simulink model "SalientPolePMSM"  (R2020b)
settings: Solver=VariableStepAuto  StartTime=0  StopTime=1  MaxStep=1e-4  RelTol=1e-4
values from neighbouring files (symbols this model uses):
  Bgain = 1    [DataSalientPolePMSM-DESKTOP-IINSHMA.m]    (also in DataSalientPolePMSM.m)
  Gcc_1ord = 1/(s/bandwidth(Gcc) + 1)    [DataSalientPolePMSM-DESKTOP-IINSHMA.m]    (also in DataSalientPolePMSM.m)
  lamdVec = mot.Ld*idVec+mot.lammg    [DataSalientPolePMSM-DESKTOP-IINSHMA.m]    (also in DataSalientPolePMSM.m)
  lamqVec = mot.Lq*iqVec    [DataSalientPolePMSM-DESKTOP-IINSHMA.m]    (also in DataSalientPolePMSM.m)
  TAB0_abc = Tabc_AB0^-1    [DataSalientPolePMSM-DESKTOP-IINSHMA.m]    (also in DataSalientPolePMSM.m)
  Tabc_AB0 = 2/3.*[     1       -1/2       -1/2 ... (first row only)    [DataSalientPolePMSM-DESKTOP-IINSHMA.m]    (also in DataSalientPolePMSM.m)
  Talphabeta_abc = Tabc_alphabeta^(-1)    [DataSalientPolePMSM-DESKTOP-IINSHMA.m]    (also in DataSalientPolePMSM.m)
undefined symbols (not defined in the file or in its folder): DiscIntNeverNeededParam, dqpll, inv, kid, kpd, magnitude, meas, mot, Obs, PI, stconv
libraries: simulink x53, pid_lib x3, powerlib x2, eeBldcCommutationLogic x1, electricdrivelib x1
(part 4 of 7)

== system SalientPolePMSM/DT SENSORLESS ALGORITHM AB/PII ==
  e : Inport
  Add : Sum  Inputs=+++
  Delay : Delay  DelayLength=1
  Delay1 : Delay  DelayLength=1
  Delay2 : Delay  DelayLength=1
  Discrete Filter1 : DiscreteFilter  Numerator=[Obs.lpf.alpha]  Denominator=[1 ((Obs.lpf.alpha)-1)]  SampleTime=Obs.Ts
  Discrete-Time Integrator : DiscreteIntegrator  SampleTime=Obs.Ts  ICPrevOutput=DiscIntNeverNeededParam  ICPrevScaledInput=DiscIntNeverNeededParam
  Gain1 : Gain  Gain=0.00001*0
  Gain6 : Gain  Gain=Obs.PI.ki*Obs.Ts*0.01
  Gain7 : Gain  Gain=Obs.PI.kp
  MATLAB Function1 : MATLAB Function  TreatAsAtomicUnit=on
  MATLAB Function2 : MATLAB Function  TreatAsAtomicUnit=on
  Sum1 : Sum  Inputs=++|
  Sum2 : Sum  Inputs=++|
  Sum3 : Sum  Inputs=++|
  w_est : Outport
  th_est : Outport  Port=2
  wires:
  Sum1/1 -> Delay/1
  Gain6/1 -> Add/1
  Delay/1 -> Gain6/1, Sum1/1
  Gain7/1 -> Add/2
  Delay1/1 -> Sum3/2, Sum2/1
  Sum2/1 -> Delay1/1
  Sum3/1 -> Delay2/1
  Delay2/1 -> Gain1/1, Sum3/1
  Gain1/1 -> Add/3
  Add/1 -> Discrete Filter1/1  "w_est"
  e/1 -> Sum2/2, Sum1/2, Gain7/1
  Discrete Filter1/1 -> Discrete-Time Integrator/1, MATLAB Function1/1(u)
  Discrete-Time Integrator/1 -> MATLAB Function2/1(u)
  MATLAB Function2/1(y) -> th_est/1
  MATLAB Function1/1(y) -> w_est/1

== system SalientPolePMSM/DT SENSORLESS ALGORITHM AB/Rev_Park + Rev_Clarke1 ==
  note: INPUTS
  Iabc : Inport
  Demux1 : Demux  Outputs=3
  Gain : Gain  Gain=sqrt(3)
  Gain1 : Gain  Gain=1/2
  Mux : Mux  Inputs=2
  Sum2 : Sum  Inputs=--|
  Terminator : Terminator
  AB : Outport
  wires:
  Demux1/3 -> Terminator/1
  Iabc/1 -> Demux1/1
  Demux1/2 -> Gain/1
  Gain/1 -> Sum2/2
  Sum2/1 -> Gain1/1
  Demux1/1 -> Mux/1, Sum2/1
  Mux/1 -> AB/1
  Gain1/1 -> Mux/2

== system SalientPolePMSM/DT SENSORLESS ALGORITHM AB/alpha axis observer ==
  u_alpha : Inport
  i_alpha_ref : Inport  Port=2
  wel_est : Inport  Port=3
  Gain : Gain  Gain=Obs.Ts/mot.Lq
  Gain1 : Gain  Gain=-mot.R*Obs.Ts/mot.Lq
  Gain2 : Gain  Gain=Obs.Lab(1)
  Gain3 : Gain  Gain=-Obs.Ts/mot.Lq
  Gain4 : Gain  Gain=Obs.Lab(2)
  Product : Product
  Sum{,1,3,5..6} (5 alike) : Sum  Inputs=|++
  Sum2 : Sum  Inputs=++|
  Sum4 : Sum  Inputs=-+|
  e_alpha(k+1) : Outport
  i_alpha(k + 1) : Outport  Port=2
  wires:
  Sum/1 -> Sum4/2, Sum/2, Gain1/1, i_alpha(k + 1)/1
  Gain/1 -> Sum3/1
  Gain1/1 -> Sum1/2
  Sum1/1 -> Sum/1
  i_alpha_ref/1 -> Sum4/1
  Sum4/1 -> Gain4/1, Gain2/1
  Gain2/1 -> Sum3/2
  Sum2/1 -> Sum1/1
  Sum3/1 -> Sum2/2
  Sum6/1 -> Gain3/1, Sum6/2, e_alpha(k+1)/1
  Gain3/1 -> Sum2/1
  Gain4/1 -> Sum5/2
  u_alpha/1 -> Product/2, Gain/1
  wel_est/1 -> Product/1
  Sum5/1 -> Sum6/1
  Product/1 -> Sum5/1

== system SalientPolePMSM/DT SENSORLESS ALGORITHM AB/alpha axis observer2 ==
  u_beta : Inport
  i_beta_ref : Inport  Port=2
  wel_est : Inport  Port=3
  Gain : Gain  Gain=Obs.Ts/mot.Lq
  Gain1 : Gain  Gain=-mot.R*Obs.Ts/mot.Lq
  Gain2 : Gain  Gain=Obs.Lab(1)
  Gain3 : Gain  Gain=-Obs.Ts/mot.Lq
  Gain4 : Gain  Gain=Obs.Lab(2)
  Product : Product
  Sum{,1,3,5..6} (5 alike) : Sum  Inputs=|++
  Sum2 : Sum  Inputs=++|
  Sum4 : Sum  Inputs=-+|
  e_beta(k+1) : Outport
  i_beta(k + 1) : Outport  Port=2
  wires:
  Sum/1 -> i_beta(k + 1)/1, Sum4/2, Sum/2, Gain1/1
  Gain/1 -> Sum3/1
  Gain1/1 -> Sum1/2
  Sum1/1 -> Sum/1
  i_beta_ref/1 -> Sum4/1
  Sum4/1 -> Gain4/1, Gain2/1
  Gain2/1 -> Sum3/2
  Sum2/1 -> Sum1/1
  Sum3/1 -> Sum2/2
  Sum5/1 -> Gain3/1, Sum5/2, e_beta(k+1)/1
  Gain3/1 -> Sum2/1
  Sum6/1 -> Sum5/1
  u_beta/1 -> Product/2, Gain/1
  Product/1 -> Sum6/1
  wel_est/1 -> Product/1
  Gain4/1 -> Sum6/2

== system SalientPolePMSM/DT SENSORLESS ALGORITHM DQ/Clarke + Park 5 ==
  note: INPUTS
  note: OUTPUT
  note: INPUTS
  abc : Inport
  thme : Inport  Port=2
  Add1 : Sum  Inputs=+-
  Add2 : Sum
  Add3 : Sum  Inputs=-+
  Add4 : Sum
  Cos1 : Trigonometry  Operator=cos
  Cos2 : Trigonometry  Operator=cos
  Demux1 : Demux  Outputs=3
  Demux2 : Demux  Outputs=3
  Demux3 : Demux  Outputs=3
  Gain : Gain  Gain=sqrt(3)
  Gain1 : Gain  Gain=Tabc_AB0  Multiplication=Matrix(K*u) (u vector)
  Gain10 : Gain  Gain=-1/sqrt(3)
  Gain2 : Gain  Gain=1/2
  Gain9 : Gain  Gain=2
  Mux : Mux  Inputs=2
  Mux1 : Mux  Inputs=2
  Mux2 : Mux  Inputs=3
  Product{,1..7} (8 alike) : Product
  Scope : Scope  NumInputPorts=2
  Sin1 : Trigonometry
  Sin2 : Trigonometry
  Sum2 : Sum  Inputs=--|
  Sum5 : Sum  Inputs=++|
  Terminator : Terminator
  Terminator1 : Terminator
  dq : Outport
  wires:
  Demux2/3 -> Terminator/1
  Product/1 -> Add2/1
  Product1/1 -> Add2/2
  Cos2/1 -> Product/2, Product3/1
  Demux2/1 -> Product3/2, Product1/1
  Product3/1 -> Add3/2
  Product2/1 -> Add3/1
  Demux2/2 -> Product2/1, Product/1
  Sin2/1 -> Product2/2, Product1/2
  Add3/1 -> Mux1/2
  Add2/1 -> Mux1/1
  Sum5/1 -> Gain10/1
  Gain9/1 -> Sum5/2
  Demux1/2 -> Gain9/1
  Demux1/3 -> Mux2/3
  Demux1/1 -> Mux2/1, Sum5/1
  Gain10/1 -> Mux2/2
  Gain1/1 -> Demux2/1, Scope/1
  Add1/1 -> Mux/1
  Sin1/1 -> Product5/2, Product4/2
  Gain/1 -> Sum2/2
  Product5/1 -> Add1/2
  Cos1/1 -> Product6/2, Product7/1
  Sum2/1 -> Gain2/1
  Demux3/1 -> Product5/1, Product6/1, Sum2/1
  Demux3/2 -> Gain/1
  Product4/1 -> Add4/2
  Product7/1 -> Add1/1
  Product6/1 -> Add4/1
  Demux3/3 -> Terminator1/1
  Add4/1 -> Mux/2
  Gain2/1 -> Product7/2, Product4/1
  thme/1 -> Sin2/1, Cos2/1
  Mux1/1 -> dq/1
  abc/1 -> Gain1/1

== system SalientPolePMSM/DT SENSORLESS ALGORITHM DQ/Classic PLL1 ==
  e_d : Inport
  e_q : Inport  Port=2
  Cos : Trigonometry  Operator=cos
  Delay{1..4} (4 alike) : Delay  DelayLength=1  SampleTime=Obs.Ts
  Discrete Filter1 : DiscreteFilter  Commented=on  Numerator=[dqpll.lpf.alpha]  Denominator=[1 (dqpll.lpf.alpha-1)]
  Discrete PID Controller : pid_lib/PID Controller  Controller=PID  Form=Parallel  TimeDomain=Discrete-time  UseExternalTs=off  SampleTime=Obs.Ts  IntegratorMethod=Forward Euler  FilterMethod=Forward Euler  ControllerParametersSource=internal  P=Obs.PI.kp*0.01  I=Obs.PI.ki*0.1  D=0  UseFilter=off  N=100  TunerSelectOption=Transfer Function Based (PID Tuner App)  ZeroCross=off  InitialConditionSource=internal  InitialConditionForIntegrator=0  InitialConditionForFilter=0  DifferentiatorICPrevScaledInput=0  ExternalReset=none  TrackingMode=off  Kt=1  LimitOutput=off  SatLimitsSource=internal  UpperSaturationLimit=inf  LowerSaturationLimit=-inf  LinearizeAsGain=off  AntiWindupMode=none  Kb=1  POutMin=[]  POutMax=[]  IOutMin=[]  IOutMax=[]  DOutMin=[]  DOutMax=[]  NOutMin=[]  NOutMax=[]  SumOutMin=[]  SumOutMax=[]  SaturationOutMin=[]  SaturationOutMax=[]  PParamMin=[]  PParamMax=[]  IParamMin=[]  IParamMax=[]  DParamMin=[]  DParamMax=[]  NParamMin=[]  NParamMax=[]  KbParamMin=[]  KbParamMax=[]  KtParamMin=[]  KtParamMax=[]  KbOutMin=[]  KbOutMax=[]  KtOutMin=[]  KtOutMax=[]  IntegratorOutMin=[]  IntegratorOutMax=[]  FilterOutMin=[]  FilterOutMax=[]  SumI1OutMin=[]  SumI1OutMax=[]  SumI2OutMin=[]  SumI2OutMax=[]  SumI3OutMin=[]  SumI3OutMax=[]  SumI4OutMin=[]  SumI4OutMax=[]  SumDOutMin=[]  SumDOutMax=[]  DifferentiatorOutMin=[]  DifferentiatorOutMax=[]  FilterDiffOutCoefMin=[]  FilterDiffOutCoefMax=[]  ReciprocalOutMin=[]  ReciprocalOutMax=[]  SumDenOutMin=[]  SumDenOutMax=[]  SumNumOutMin=[]  SumNumOutMax=[]  DivideOutMin=[]  DivideOutMax=[]  UdiffTsProdOutMin=[]  UdiffTsProdOutMax=[]  NTsProdOutMin=[]  NTsProdOutMax=[]  UintegralTsProdOutMin=[]  UintegralTsProdOutMax=[]  UngainTsProdOutMin=[]  UngainTsProdOutMax=[]  IntegratorContinuousStateAttributes=''  IntegratorStateMustResolveToSignalObject=off  IntegratorRTWStateStorageClass=Auto  FilterContinuousStateAttributes=''  FilterStateMustResolveToSignalObject=off  FilterRTWStateStorageClass=Auto  ParallelPVariant=InternalParameters  IdealPVariant=Disabled  IVariant=InternalParameters  DVariant=InternalParameters  IntegratorVariant=Discrete  SatVariant=Disabled  AWVariant=Passthrough  PCopyVariant=Disabled  TRVariant=Disabled  FdbkBlocksVariant=Forward  IdealPFdbkVariant=Disabled  SatFdbkVariant=Disabled  DerivativeFilterVariant=Differentiator  NVariant=Passthrough  NCopyVariant=Disabled_SignalSpec  FilterICVariant=InternalICsDifferentiator  IntegratorICVariant=InternalICs  ExternalResetVariant=Disabled  TRSumVariant=Passthrough  SumFdbkVariant=Disabled  SumVariant=Sum_PID  TsampFilterVariant=InternalTs  TsampNgainVariant=Passthrough  TsampIntegralVariant=Passthrough  ExternalSaturationOutDataTypeStr=Inherit: Same as second input
  Discrete-Time Integrator : DiscreteIntegrator  gainval=1  SampleTime=Obs.Ts  ICPrevOutput=DiscIntNeverNeededParam  ICPrevScaledInput=DiscIntNeverNeededParam
  Divide1 : Product  Inputs=**
  Divide2 : Product  Inputs=**
  Gain : Gain
  MATLAB Function1 : MATLAB Function  TreatAsAtomicUnit=on
  Scope : Scope  NumInputPorts=2
  Scope1 : Scope  NumInputPorts=2
  Sin : Trigonometry
  Sum : Sum  Inputs=-|+
  thme_est1 : Outport
  wme_est1 : Outport  Port=2
  wires:
  e_q/1 -> Delay1/1
  e_d/1 -> Delay2/1
  Delay2/1 -> Divide1/1
  Divide1/1 -> Scope/1, Sum/1
  Divide2/1 -> Scope/2, Sum/2
  Delay1/1 -> Divide2/1
  Sin/1 -> Divide2/2
  Cos/1 -> Divide1/2
  Delay4/1 -> Sin/1
  Delay3/1 -> Cos/1
  Discrete-Time Integrator/1 -> Delay4/1, thme_est1/1, Delay3/1
  Sum/1 -> Discrete PID Controller/1, Scope1/1
  Gain/1 -> wme_est1/1
  Discrete PID Controller/1 -> Gain/1, Discrete-Time Integrator/1

== system SalientPolePMSM/DT SENSORLESS ALGORITHM DQ/DECOUPLING ==
  note: OUTPUTS:
  note: INPUTS:
  idq_est : Inport
  udq_est : Inport  Port=2
  wme_est : Inport  Port=3
  Demux1 : Demux  Outputs=2
  Demux2 : Demux  Outputs=2
  Gain10 : Gain  Gain=dqpll.Lq
  Gain11 : Gain  Gain=dqpll.Lq
  Mux : Mux  Inputs=2
  Mux1 : Mux  Inputs=2
  Product : Product
  Product1 : Product
  Sum1 : Sum  Inputs=-+|
  Sum3 : Sum  Inputs=++|
  ud' id : Outport
  uq' iq : Outport  Port=2
  wires:
  Sum1/1 -> Mux1/1
  Product/1 -> Gain10/1
  Product1/1 -> Gain11/1
  Gain10/1 -> Sum3/1
  Gain11/1 -> Sum1/1
  Sum3/1 -> Mux/1
  idq_est/1 -> Demux2/1
  udq_est/1 -> Demux1/1
  Mux1/1 -> uq' iq/1
  Mux/1 -> ud' id/1
  wme_est/1 -> [WME_EST]
  [WME_EST] -> Product1/2
  [WME_EST] -> Product/1
  Demux2/2 -> [IQ]
  [IQ] -> Product/2
  [IQ] -> Mux1/2
  Demux2/1 -> [ID]
  [ID] -> Mux/2
  [ID] -> Product1/1
  Demux1/1 -> [UD]
  Demux1/2 -> [UQ]
  [UD] -> Sum3/2
  [UQ] -> Sum1/2

== system SalientPolePMSM/DT SENSORLESS ALGORITHM DQ/Normalized and improved PLL3 ==
  e_d : Inport
  e_q : Inport  Port=2
  Cos : Trigonometry  Operator=cos
  Delay{1..3,5} (4 alike) : Delay  DelayLength=1  SampleTime=100e-6
  Discrete Filter1 : DiscreteFilter  Commented=on  Numerator=[dqpll.lpf.alpha]  Denominator=[1 (dqpll.lpf.alpha-1)]
  Discrete PI : Subsystem
  Discrete-Time Integrator : DiscreteIntegrator  SampleTime=100e-6  ICPrevOutput=DiscIntNeverNeededParam  ICPrevScaledInput=DiscIntNeverNeededParam
  Divide1 : Product  Inputs=**
  Divide2 : Product  Inputs=**
  Divide3 : Product  Inputs=**
  Gain : Gain  Gain=-2
  Gain1 : Gain  Gain=0.5
  Gain2 : Gain  Gain=2
  Gain3 : Gain  Gain=2
  Gain4 : Gain
  Power of 1 : Math  Operator=magnitude^2  SaturateOnIntegerOverflow=on
  Power of 10 : Math  Operator=magnitude^2  SaturateOnIntegerOverflow=on
  Scope : Scope  NumInputPorts=2
  Sin : Trigonometry
  Sum : Sum  Inputs=-|-
  Sum1 : Sum  Inputs=|+-
  thme_est1 : Outport
  wme_est1 : Outport  Port=2
  wires:
  Divide1/1 -> Scope/1, Sum/1
  Divide2/1 -> Scope/2, Sum/2
  Sin/1 -> Divide2/2
  Cos/1 -> Divide1/2
  Discrete-Time Integrator/1 -> thme_est1/1, Delay5/1, Delay2/1
  Discrete PI/1(w_est) -> Gain4/1, Discrete-Time Integrator/1
  Gain/1 -> Divide3/1
  Divide3/1 -> Divide2/1
  Power of 1/1 -> Sum1/1
  Power of 10/1 -> Sum1/2
  Sum1/1 -> Divide1/1
  Sum/1 -> Gain1/1
  Gain1/1 -> Discrete PI/1(e)
  Gain3/1 -> Sin/1
  Gain2/1 -> Cos/1
  Delay1/1 -> Power of 1/1, Gain/1
  e_d/1 -> Delay1/1
  e_q/1 -> Delay3/1
  Delay3/1 -> Divide3/2, Power of 10/1
  Delay5/1 -> Gain3/1
  Delay2/1 -> Gain2/1
  Gain4/1 -> wme_est1/1

== system SalientPolePMSM/DT SENSORLESS ALGORITHM DQ/PII ==
  theta(k+1) : Inport
  theta(k) : Inport  Port=2
  Add : Sum  Inputs=+++
  Delay : Delay  DelayLength=1
  Delay1 : Delay  DelayLength=1
  Delay2 : Delay  DelayLength=1
  Gain1 : Gain  Gain=0.002*0
  Gain6 : Gain  Gain=5
  Gain7 : Gain  Gain=1600
  Sum : Sum  Inputs=|+-
  Sum1 : Sum  Inputs=++|
  Sum2 : Sum  Inputs=++|
  Sum3 : Sum  Inputs=++|
  w_est : Outport
  wires:
  Sum1/1 -> Delay/1
  Gain6/1 -> Add/1
  Delay/1 -> Gain6/1, Sum1/1
  Add/1 -> w_est/1  "w_est"
  Gain7/1 -> Add/2
  Delay1/1 -> Sum3/2, Sum2/1
  Sum2/1 -> Delay1/1
  Sum3/1 -> Delay2/1
  Delay2/1 -> Gain1/1, Sum3/1
  Gain1/1 -> Add/3
  theta(k+1)/1 -> Sum/1
  Sum/1 -> Sum1/2, Sum2/2, Gain7/1

== system SalientPolePMSM/DT SENSORLESS ALGORITHM DQ/Rev_Park + Rev_Clarke1 ==
  note: INPUTS
  Iabc : Inport
  thme1 : Inport  Port=2
  Add1 : Sum  Inputs=+-
  Add4 : Sum
  Cos1 : Trigonometry  Operator=cos
  Demux1 : Demux  Outputs=3
  Gain : Gain  Gain=sqrt(3)
  Gain1 : Gain  Gain=1/2
  Mux : Mux  Inputs=2
  Product{4..7} (4 alike) : Product
  Sin1 : Trigonometry
  Sum2 : Sum  Inputs=--|
  Terminator : Terminator
  dq : Outport
  wires:
  Demux1/3 -> Terminator/1
  Iabc/1 -> Demux1/1
  Cos1/1 -> Product6/2, Product7/1
  Product5/1 -> Add1/2
  Sin1/1 -> Product5/2, Product4/2
  Product6/1 -> Add4/1
  thme1/1 -> Sin1/1, Cos1/1
  Product4/1 -> Add4/2
  Product7/1 -> Add1/1
  Demux1/2 -> Gain/1
  Gain/1 -> Sum2/2
  Sum2/1 -> Gain1/1
  Gain1/1 -> Product7/2, Product4/1
  Demux1/1 -> Product5/1, Product6/1, Sum2/1
  Mux/1 -> dq/1
  Add1/1 -> Mux/1
  Add4/1 -> Mux/2

== system SalientPolePMSM/Discrete SS ALGORITHM/DECOUPLING ==
  note: OUTPUTS:
  note: INPUTS:
  idq_est : Inport
  udq_est : Inport  Port=2
  wme_est : Inport  Port=3
  Demux1 : Demux  Outputs=2
  Demux2 : Demux  Outputs=2
  Gain10 : Gain  Gain=dqpll.Lq
  Gain11 : Gain  Gain=dqpll.Lq
  Mux : Mux  Inputs=2
  Mux1 : Mux  Inputs=2
  Product : Product
  Product1 : Product
  Sum1 : Sum  Inputs=-+|
  Sum3 : Sum  Inputs=++|
  ud' id : Outport
  uq' iq : Outport  Port=2
  wires:
  Sum1/1 -> Mux1/1
  Product/1 -> Gain10/1
  Product1/1 -> Gain11/1
  Gain10/1 -> Sum3/1
  Gain11/1 -> Sum1/1
  Sum3/1 -> Mux/1
  idq_est/1 -> Demux2/1
  udq_est/1 -> Demux1/1
  Mux1/1 -> uq' iq/1
  Mux/1 -> ud' id/1
  wme_est/1 -> [WME_EST]
  [WME_EST] -> Product1/2
  [WME_EST] -> Product/1
  Demux2/2 -> [IQ]
  [IQ] -> Product/2
  [IQ] -> Mux1/2
  Demux2/1 -> [ID]
  [ID] -> Mux/2
  [ID] -> Product1/1
  Demux1/1 -> [UD]
  Demux1/2 -> [UQ]
  [UD] -> Sum3/2
  [UQ] -> Sum1/2

== system SalientPolePMSM/Discrete SS ALGORITHM/PI ==
  e : Inport
  Delay : Delay  DelayLength=1
  Gain6 : Gain  Gain=dqpll.PI.ki*dqpll.Ts*10
  Gain7 : Gain  Gain=dqpll.PI.kp*2
  Sum1 : Sum  Inputs=++|
  Sum2 : Sum  Inputs=++|
  w_est : Outport
  wires:
  Gain7/1 -> Sum2/2
  Sum2/1 -> w_est/1  "w_est"
  e/1 -> Sum1/2, Gain7/1
  Delay/1 -> Sum1/1, Gain6/1
  Gain6/1 -> Sum2/1
  Sum1/1 -> Delay/1

== system SalientPolePMSM/Discrete SS ALGORITHM/PII ==
  e : Inport
  Add : Sum  Inputs=+++
  Delay : Delay  DelayLength=1
  Delay1 : Delay  DelayLength=1
  Delay2 : Delay  DelayLength=1
  Gain1 : Gain  Gain=dqpll.PI.k3*dqpll.Ts^2
  Gain6 : Gain  Gain=dqpll.PI.k2*dqpll.Ts
  Gain7 : Gain  Gain=dqpll.PI.k1
  Sum1 : Sum  Inputs=++|
  Sum2 : Sum  Inputs=++|
  Sum3 : Sum  Inputs=++|
  w_est : Outport
  wires:
  Sum1/1 -> Delay/1
  Gain6/1 -> Add/1
  Delay/1 -> Gain6/1, Sum1/1
  Add/1 -> w_est/1  "w_est"
  Gain7/1 -> Add/2
  e/1 -> Sum2/2, Sum1/2, Gain7/1
  Delay1/1 -> Sum3/2, Sum2/1
  Sum2/1 -> Delay1/1
  Sum3/1 -> Delay2/1
  Delay2/1 -> Gain1/1, Sum3/1
  Gain1/1 -> Add/3

== system SalientPolePMSM/Discrete SS ALGORITHM/Subsystem5 ==
  note: OUTPUT
  note: INPUTS
  abc : Inport
  thme : Inport  Port=2
  Add2 : Sum
  Add3 : Sum  Inputs=-+
  Cos2 : Trigonometry  Operator=cos
  Demux2 : Demux  Outputs=3
  Gain : Gain  Gain=Tabc_AB0  Multiplication=Matrix(K*u) (u vector)
  Mux1 : Mux  Inputs=2
  Product{,1..3} (4 alike) : Product
  Sin2 : Trigonometry
  Terminator : Terminator
  dq : Outport
  wires:
  Mux1/1 -> dq/1
  Sin2/1 -> Product1/2, Product2/2
  Demux2/2 -> Product3/2, Product1/1
  Product2/1 -> Add3/1
  Product3/1 -> Add3/2
  thme/1 -> Sin2/1, Cos2/1
  Demux2/1 -> Product2/1, Product/1
  Cos2/1 -> Product3/1, Product/2
  Product1/1 -> Add2/2
  Add3/1 -> Mux1/2
  Add2/1 -> Mux1/1
  Product/1 -> Add2/1
  Gain/1 -> Demux2/1  "AB0"
  Demux2/3 -> Terminator/1
  abc/1 -> Gain/1

== system SalientPolePMSM/Discrete SS ALGORITHM/Subsystem6 ==
  note: INPUTS
  note: OUTPUT
  abc : Inport
  thme : Inport  Port=2
  Add2 : Sum
  Add3 : Sum  Inputs=-+
  Cos2 : Trigonometry  Operator=cos
  Demux2 : Demux  Outputs=3
  Gain : Gain  Gain=Tabc_AB0  Multiplication=Matrix(K*u) (u vector)
  Mux1 : Mux  Inputs=2
  Product{,1..3} (4 alike) : Product
  Sin2 : Trigonometry
  Terminator : Terminator
  dq : Outport
  wires:
  abc/1 -> Gain/1
  Demux2/3 -> Terminator/1
  Gain/1 -> Demux2/1  "AB0"
  Product/1 -> Add2/1
  Add2/1 -> Mux1/1
  Add3/1 -> Mux1/2
  Product1/1 -> Add2/2
  Cos2/1 -> Product/2, Product3/1
  Demux2/1 -> Product/1, Product2/1
  thme/1 -> Cos2/1, Sin2/1
  Product3/1 -> Add3/2
  Product2/1 -> Add3/1
  Demux2/2 -> Product1/1, Product3/2
  Sin2/1 -> Product2/2, Product1/2
  Mux1/1 -> dq/1

== system SalientPolePMSM/Discrete SS ALGORITHM1/DECOUPLING ==
  note: OUTPUTS:
  note: INPUTS:
  idq_est : Inport
  udq_est : Inport  Port=2
  wme_est : Inport  Port=3
  Demux1 : Demux  Outputs=2
  Demux2 : Demux  Outputs=2
  Gain10 : Gain  Gain=dqpll.Lq
  Gain11 : Gain  Gain=dqpll.Lq
  Mux : Mux  Inputs=2
  Mux1 : Mux  Inputs=2
  Product : Product
  Product1 : Product
  Sum1 : Sum  Inputs=-+|
  Sum3 : Sum  Inputs=++|
  ud' id : Outport
  uq' iq : Outport  Port=2
  wires:
  Sum1/1 -> Mux1/1
  Product/1 -> Gain10/1
  Product1/1 -> Gain11/1
  Gain10/1 -> Sum3/1
  Gain11/1 -> Sum1/1
  Sum3/1 -> Mux/1
  idq_est/1 -> Demux2/1
  udq_est/1 -> Demux1/1
  Mux1/1 -> uq' iq/1
  Mux/1 -> ud' id/1
  wme_est/1 -> [WME_EST]
  [WME_EST] -> Product1/2
  [WME_EST] -> Product/1
  Demux2/2 -> [IQ]
  [IQ] -> Product/2
  [IQ] -> Mux1/2
  Demux2/1 -> [ID]
  [ID] -> Mux/2
  [ID] -> Product1/1
  Demux1/1 -> [UD]
  Demux1/2 -> [UQ]
  [UD] -> Sum3/2
  [UQ] -> Sum1/2

== system SalientPolePMSM/Discrete SS ALGORITHM1/PI ==
  e : Inport
  Delay : Delay  DelayLength=1
  Gain6 : Gain  Gain=dqpll.PI.ki*dqpll.Ts
  Gain7 : Gain  Gain=dqpll.PI.kp
  Sum1 : Sum  Inputs=++|
  Sum2 : Sum  Inputs=++|
  w_est : Outport
  wires:
  Gain7/1 -> Sum2/2
  Sum2/1 -> w_est/1  "w_est"
  e/1 -> Sum1/2, Gain7/1
  Delay/1 -> Sum1/1, Gain6/1
  Gain6/1 -> Sum2/1
  Sum1/1 -> Delay/1

== system SalientPolePMSM/Discrete SS ALGORITHM1/PII ==
  e : Inport
  Add : Sum  Inputs=+++
  Delay : Delay  DelayLength=1
  Delay1 : Delay  DelayLength=1
  Delay2 : Delay  DelayLength=1
  Gain1 : Gain  Gain=dqpll.PI.k3*dqpll.Ts^2
  Gain6 : Gain  Gain=dqpll.PI.k2*dqpll.Ts
  Gain7 : Gain  Gain=dqpll.PI.k1
  Sum1 : Sum  Inputs=++|
  Sum2 : Sum  Inputs=++|
  Sum3 : Sum  Inputs=++|
  w_est : Outport
  wires:
  Sum1/1 -> Delay/1
  Gain6/1 -> Add/1
  Delay/1 -> Gain6/1, Sum1/1
  Add/1 -> w_est/1  "w_est"
  Gain7/1 -> Add/2
  e/1 -> Sum2/2, Sum1/2, Gain7/1
  Delay1/1 -> Sum3/2, Sum2/1
  Sum2/1 -> Delay1/1
  Sum3/1 -> Delay2/1
  Delay2/1 -> Gain1/1, Sum3/1
  Gain1/1 -> Add/3

== system SalientPolePMSM/Discrete SS ALGORITHM1/Subsystem5 ==
  note: OUTPUT
  note: INPUTS
  abc : Inport
  thme : Inport  Port=2
  Add2 : Sum
  Add3 : Sum  Inputs=-+
  Cos2 : Trigonometry  Operator=cos
  Demux2 : Demux  Outputs=3
  Gain : Gain  Gain=Tabc_AB0  Multiplication=Matrix(K*u) (u vector)
  Mux1 : Mux  Inputs=2
  Product{,1..3} (4 alike) : Product
  Sin2 : Trigonometry
  Terminator : Terminator
  dq : Outport
  wires:
  Mux1/1 -> dq/1
  Sin2/1 -> Product1/2, Product2/2
  Demux2/2 -> Product3/2, Product1/1
  Product2/1 -> Add3/1
  Product3/1 -> Add3/2
  thme/1 -> Sin2/1, Cos2/1
  Demux2/1 -> Product2/1, Product/1
  Cos2/1 -> Product3/1, Product/2
  Product1/1 -> Add2/2
  Add3/1 -> Mux1/2
  Add2/1 -> Mux1/1
  Product/1 -> Add2/1
  Gain/1 -> Demux2/1  "AB0"
  Demux2/3 -> Terminator/1
  abc/1 -> Gain/1

== system SalientPolePMSM/Discrete SS ALGORITHM1/Subsystem6 ==
  note: INPUTS
  note: OUTPUT
  abc : Inport
  thme : Inport  Port=2
  Add2 : Sum
  Add3 : Sum  Inputs=-+
  Cos2 : Trigonometry  Operator=cos
  Demux2 : Demux  Outputs=3
  Gain : Gain  Gain=Tabc_AB0  Multiplication=Matrix(K*u) (u vector)
  Mux1 : Mux  Inputs=2
  Product{,1..3} (4 alike) : Product
  Sin2 : Trigonometry
  Terminator : Terminator
  dq : Outport
  wires:
  abc/1 -> Gain/1
  Demux2/3 -> Terminator/1
  Gain/1 -> Demux2/1  "AB0"
  Product/1 -> Add2/1
  Add2/1 -> Mux1/1
  Add3/1 -> Mux1/2
  Product1/1 -> Add2/2
  Cos2/1 -> Product/2, Product3/1
  Demux2/1 -> Product/1, Product2/1
  thme/1 -> Cos2/1, Sin2/1
  Product3/1 -> Add3/2
  Product2/1 -> Add3/1
  Demux2/2 -> Product1/1, Product3/2
  Sin2/1 -> Product2/2, Product1/2
  Mux1/1 -> dq/1

== system SalientPolePMSM/FOC1/Changed1 ==
  note: Variations
  note: INPUTS
  note: OUTPUT
  dq : Inport
  thme : Inport  Port=2
  Add2 : Sum
  Add3 : Sum  Inputs=+-
  Cos2 : Trigonometry  Operator=cos
  Demux2 : Demux  Outputs=2
  Mux1 : Mux  Inputs=2
  Product{,1..3} (4 alike) : Product
  Sin2 : Trigonometry
  Subsystem : Subsystem
  AB : Outport
  wires:
  Product3/1 -> Add2/1
  Demux2/2 -> Product2/1, Product3/2
  Demux2/1 -> Product/1, Product1/1
  Mux1/1 -> AB/1
  Sin2/1 -> Product1/2, Product2/2
  thme/1 -> Sin2/1, Cos2/1
  Cos2/1 -> Product3/1, Product/2
  Product1/1 -> Add2/2
  dq/1 -> Demux2/1
  Add3/1 -> Mux1/2
  Add2/1 -> Mux1/1
  Product2/1 -> Add3/2
  Product/1 -> Add3/1

== system SalientPolePMSM/FOC1/Circle Limitation ==
  dq : Inport
  Demux : Demux  Outputs=2
  Gain : Gain  Gain=1000
  Gain1 : Gain  Gain=1000
  Gain2 : Gain  Gain=1/1000
  Gain3 : Gain  Gain=1/1000
  MATLAB Function : MATLAB Function  TreatAsAtomicUnit=on
  Mux : Mux  Inputs=2
  dq* : Outport
  wires:
  Demux/2 -> Gain1/1
  Demux/1 -> Gain/1
  Mux/1 -> dq*/1
  dq/1 -> Demux/1
  MATLAB Function/1(new_d) -> Gain2/1
  MATLAB Function/2(new_q) -> Gain3/1
  Gain2/1 -> Mux/1
  Gain3/1 -> Mux/2
  Gain/1 -> MATLAB Function/1(u_d)
  Gain1/1 -> MATLAB Function/2(u_q)

== system SalientPolePMSM/FOC1/Decoupling1 ==
  note: INPUTS:
  note: OUTPUT:
  udq* : Inport
  idq : Inport  Port=2
  wme : Inport  Port=3
  Demux : Demux  Outputs=2
  Demux1 : Demux  Outputs=2
  Demux2 : Demux  Outputs=2
  Gain : Gain  Gain=PI.cur.Ld
  Gain1 : Gain  Gain=PI.cur.Lq
  Gain2 : Gain  Gain=PI.cur.lammg
  Mux : Mux  Inputs=2
  Product : Product
  Product1 : Product
  Scope : Scope
  Scope1 : Scope
  Subtract : Sum  Inputs=-+
  Subtract1 : Sum  Inputs=+++
  Terminator1 : Terminator
  Terminator4 : Terminator
  idq1 : InportShadow  Port=2
  wme1 : InportShadow  Port=3
  udq** : Outport
  wires:
  Product1/1 -> Scope/1, Subtract/1  "wme*iq*Lq"
  wme1/1 -> Gain1/1
  Gain1/1 -> Product1/2
  Demux1/1 -> Terminator4/1
  idq1/1 -> Demux1/1
  Demux1/2 -> Product1/1  "iq"
  udq*/1 -> Demux/1
  Mux/1 -> udq**/1
  Gain/1 -> Product/1
  Gain2/1 -> Subtract1/2  "wme*lammg"
  Subtract1/1 -> Mux/2
  wme/1 -> Gain2/1, Gain/1
  Demux/1 -> Subtract/2
  Demux2/2 -> Terminator1/1
  Demux/2 -> Subtract1/1
  Subtract/1 -> Mux/1
  Product/1 -> Subtract1/3  "wme*id*Ld"
  idq/1 -> Demux2/1, Scope1/1
  Demux2/1 -> Product/2  "id"

== system SalientPolePMSM/FOC1/Decoupling2 ==
  note: INPUTS:
  note: OUTPUT:
  udq* : Inport
  idq : Inport  Port=2
  wme : Inport  Port=3
  Demux : Demux  Outputs=2
  Demux1 : Demux  Outputs=2
  Demux2 : Demux  Outputs=2
  Gain : Gain  Gain=PI.cur.Ld
  Gain1 : Gain  Gain=PI.cur.Lq
  Gain2 : Gain  Gain=PI.cur.lammg
  Mux : Mux  Inputs=2
  Product : Product
  Product1 : Product
  Scope : Scope
  Scope1 : Scope
  Subtract : Sum  Inputs=-+
  Subtract1 : Sum  Inputs=+++
  Terminator1 : Terminator
  Terminator4 : Terminator
  idq1 : InportShadow  Port=2
  wme1 : InportShadow  Port=3
  udq** : Outport
  wires:
  Product1/1 -> Scope/1, Subtract/1  "wme*iq*Lq"
  wme1/1 -> Gain1/1
  Gain1/1 -> Product1/2
  Demux1/1 -> Terminator4/1
  idq1/1 -> Demux1/1
  Demux1/2 -> Product1/1  "iq"
  udq*/1 -> Demux/1
  Mux/1 -> udq**/1
  Gain/1 -> Product/1
  Gain2/1 -> Subtract1/2  "wme*lammg"
  Subtract1/1 -> Mux/2
  wme/1 -> Gain2/1, Gain/1
  Demux/1 -> Subtract/2
  Demux2/2 -> Terminator1/1
  Demux/2 -> Subtract1/1
  Subtract/1 -> Mux/1
  Product/1 -> Subtract1/3  "wme*id*Ld"
  idq/1 -> Demux2/1, Scope1/1
  Demux2/1 -> Product/2  "id"

== system SalientPolePMSM/FOC1/INVERTER1 ==
  note: OUTPUTS:
  note: INPUTS:
  uAB : Inport
  uBus : Inport  Port=2
  iabc : Inport  Port=3
  INVERTER power driver : Subsystem
  SVM algorithm : Subsystem
  Scope : Scope
  uabc_n* : Outport
  uabc_n*nonideal : Outport  Port=2
  satON : Outport  Port=3
  wires:
  INVERTER power driver/1(uabc_n*) -> uabc_n*/1
  uAB/1 -> SVM algorithm/1(UABref)
  INVERTER power driver/2(uabc_n*nonideal) -> uabc_n*nonideal/1
  iabc/1 -> INVERTER power driver/3(iabc)
  SVM algorithm/1(duties) -> INVERTER power driver/1(duties), Scope/1  "duties"
  [satON] -> satON/1
  SVM algorithm/2(satON) -> [satON]
  uBus/1 -> INVERTER power driver/2(uBus), SVM algorithm/2(uBus)

== system SalientPolePMSM/FOC1/INVERTER2 ==
  note: OUTPUTS:
  note: INPUTS:
  uAB : Inport
  uBus : Inport  Port=2
  iabc : Inport  Port=3
  INVERTER power driver : Subsystem
  SVM algorithm : Subsystem
  Scope : Scope  NumInputPorts=2
  Scope1 : Scope
  uabc_n* : Outport
  uabc_n*nonideal : Outport  Port=2
  satON : Outport  Port=3
  wires:
  INVERTER power driver/2(uabc_n*nonideal) -> uabc_n*nonideal/1
  iabc/1 -> INVERTER power driver/3(iabc)
  SVM algorithm/1(duties) -> Scope/1, INVERTER power driver/1(duties)  "duties"
  [satON] -> satON/1
  uBus/1 -> INVERTER power driver/2(uBus), SVM algorithm/2(uBus)
  uAB/1 -> Scope1/1, SVM algorithm/1(VABref)
  INVERTER power driver/1(uabc_n*) -> Scope/2, uabc_n*/1

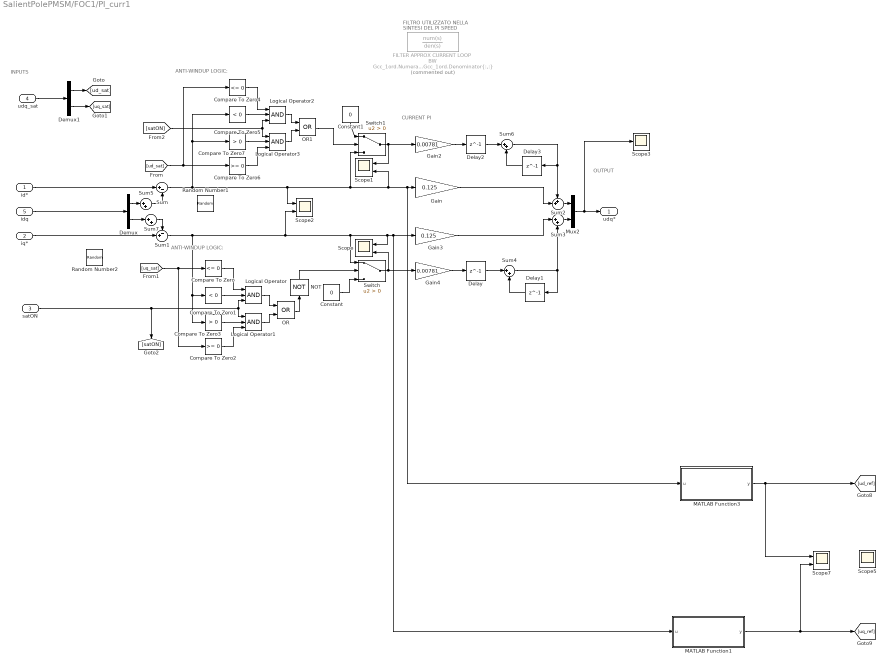
== system SalientPolePMSM/FOC1/PI_curr1 ==
  note: INPUTS
  note: OUTPUT
  note: ANTI-WINDUP LOGIC:
  note: ANTI-WINDUP LOGIC:
  note: CURRENT PI
  note: FILTRO UTILIZZATO
      | NELLA SINTESI DEL
      | PI SPEED
  id* : Inport
  iq* : Inport  Port=2
  satON : Inport  Port=3
  udq_sat : Inport  Port=4
  idq : Inport  Port=5
  Compare To Zero : simulink/Logic and Bit Operations/Compare To Zero  relop=<=  OutDataTypeStr=boolean  ZeroCross=off
  Compare To Zero1 : simulink/Logic and Bit Operations/Compare To Zero  relop=<  OutDataTypeStr=boolean  ZeroCross=off
  Compare To Zero2 : simulink/Logic and Bit Operations/Compare To Zero  relop=>=  OutDataTypeStr=boolean  ZeroCross=off
  Compare To Zero3 : simulink/Logic and Bit Operations/Compare To Zero  relop=>  OutDataTypeStr=boolean  ZeroCross=off
  Compare To Zero4 : simulink/Logic and Bit Operations/Compare To Zero  relop=<=  OutDataTypeStr=boolean  ZeroCross=off
  Compare To Zero5 : simulink/Logic and Bit Operations/Compare To Zero  relop=<  OutDataTypeStr=boolean  ZeroCross=off
  Compare To Zero6 : simulink/Logic and Bit Operations/Compare To Zero  relop=>=  OutDataTypeStr=boolean  ZeroCross=off
  Compare To Zero7 : simulink/Logic and Bit Operations/Compare To Zero  relop=>  OutDataTypeStr=boolean  ZeroCross=off
  Constant : Constant  Value=0
  Constant1 : Constant  Value=0
  Delay{,1..3} (4 alike) : Delay  DelayLength=1  SampleTime=PI.cur.Ts
  Demux : Demux  Outputs=2
  Demux1 : Demux  Outputs=2
  FILTER APPROX CURRENT LOOP BW : TransferFcn  Commented=on  Numerator=Gcc_1ord.Numerator{:,:}  Denominator=Gcc_1ord.Denominator{:,:}
  Gain : Gain  Gain=0.125
  Gain2 : Gain  Gain=0.00781
  Gain3 : Gain  Gain=0.125
  Gain4 : Gain  Gain=0.00781
  Logical Operator{,1..3} (4 alike) : Logic  Inputs=3  AllPortsSameDT=off  OutDataTypeStr=boolean
  MATLAB Function1 : MATLAB Function  TreatAsAtomicUnit=on
  MATLAB Function3 : MATLAB Function  TreatAsAtomicUnit=on
  Mux2 : Mux  Inputs=2
  NOT : Logic  Operator=NOT  AllPortsSameDT=off  OutDataTypeStr=boolean
  OR : Logic  Operator=OR  AllPortsSameDT=off  OutDataTypeStr=boolean
  OR1 : Logic  Operator=OR  AllPortsSameDT=off  OutDataTypeStr=boolean
  Random Number1 : RandomNumber  Variance=0.01  SampleTime=inv.Ts
  Random Number2 : RandomNumber  Variance=0.125  SampleTime=inv.Ts
  Scope{,1..2,7} (4 alike) : Scope  NumInputPorts=2
  Scope3 : Scope
  Scope5 : Scope
  Sum : Sum  Inputs=|+-
  Sum1 : Sum  Inputs=-+|
  Sum2 : Sum  Inputs=++|
  Sum{3..7} (5 alike) : Sum  Inputs=|++
  Switch : Switch  Criteria=u2 > Threshold
  Switch1 : Switch  Criteria=u2 > Threshold
  udq* : Outport
  wires:
  Sum/1 -> Compare To Zero5/1, Compare To Zero7/1, Switch1/3, Gain/1, MATLAB Function3/1(u), Scope1/2, Scope2/1
  Switch/1 -> Gain4/1, Scope/2
  MATLAB Function1/1(y) -> Scope7/2, [uq_ref]
  MATLAB Function3/1(y) -> [ud_ref], Scope7/1
  Sum7/1 -> Sum1/1
  Demux/2 -> Sum7/1
  Demux/1 -> Sum5/1
  Sum5/1 -> Sum/2
  Gain2/1 -> Delay2/1
  Sum6/1 -> Sum2/1, Delay3/1
  Delay2/1 -> Sum6/1
  Delay3/1 -> Sum6/2
  Delay1/1 -> Sum4/2
  Delay/1 -> Sum4/1
  iq*/1 -> Sum1/2
  Demux1/2 -> [uq_sat]
  Demux1/1 -> [ud_sat]
  udq_sat/1 -> Demux1/1
  Switch1/1 -> Gain2/1, Scope1/1
  Constant1/1 -> Switch1/1
  OR1/1 -> Switch1/2
  [satON] -> Logical Operator3/1, Logical Operator2/3
  Logical Operator2/1 -> OR1/1
  Logical Operator3/1 -> OR1/2
  Compare To Zero5/1 -> Logical Operator2/2
  Compare To Zero4/1 -> Logical Operator2/1
  Compare To Zero6/1 -> Logical Operator3/3
  [ud_sat] -> Compare To Zero6/1, Compare To Zero4/1
  Compare To Zero7/1 -> Logical Operator3/2
  Compare To Zero3/1 -> Logical Operator1/2
  [uq_sat] -> Compare To Zero/1, Compare To Zero2/1
  Compare To Zero2/1 -> Logical Operator1/3
  Compare To Zero/1 -> Logical Operator/1
  Compare To Zero1/1 -> Logical Operator/2
  Logical Operator1/1 -> OR/2
  Logical Operator/1 -> OR/1
  satON/1 -> Logical Operator1/1, Logical Operator/3, [satON]
  NOT/1 -> Switch/2
  OR/1 -> NOT/1
  Constant/1 -> Switch/3
  id*/1 -> Sum/1
  idq/1 -> Demux/1
  Gain3/1 -> Sum3/1
  Gain4/1 -> Delay/1
  Gain/1 -> Sum2/2
  Sum1/1 -> Compare To Zero1/1, Compare To Zero3/1, Gain3/1, MATLAB Function1/1(u), Scope/1, Switch/1, Scope2/2
  Sum4/1 -> Sum3/2, Delay1/1
  Sum2/1 -> Mux2/1
  Sum3/1 -> Mux2/2
  Mux2/1 -> udq*/1, Scope3/1

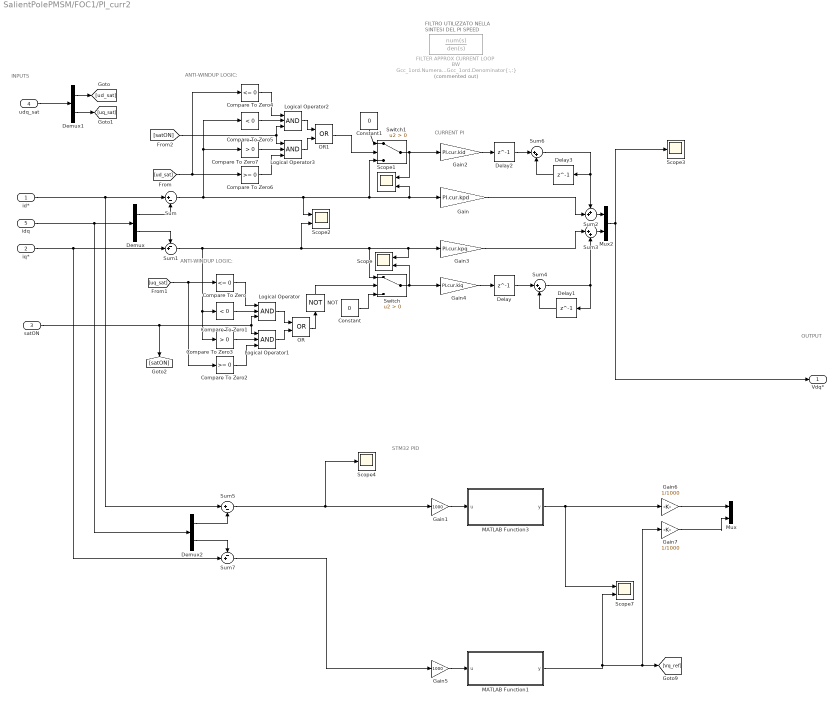
== system SalientPolePMSM/FOC1/PI_curr2 ==
  note: INPUTS
  note: OUTPUT
  note: ANTI-WINDUP LOGIC:
  note: ANTI-WINDUP LOGIC:
  note: STM32 PID
  note: FILTRO UTILIZZATO
      | NELLA SINTESI DEL
      | PI SPEED
  note: CURRENT PI
  id* : Inport
  iq* : Inport  Port=2
  satON : Inport  Port=3
  udq_sat : Inport  Port=4
  idq : Inport  Port=5
  Compare To Zero : simulink/Logic and Bit Operations/Compare To Zero  relop=<=  OutDataTypeStr=boolean  ZeroCross=off
  Compare To Zero1 : simulink/Logic and Bit Operations/Compare To Zero  relop=<  OutDataTypeStr=boolean  ZeroCross=off
  Compare To Zero2 : simulink/Logic and Bit Operations/Compare To Zero  relop=>=  OutDataTypeStr=boolean  ZeroCross=off
  Compare To Zero3 : simulink/Logic and Bit Operations/Compare To Zero  relop=>  OutDataTypeStr=boolean  ZeroCross=off
  Compare To Zero4 : simulink/Logic and Bit Operations/Compare To Zero  relop=<=  OutDataTypeStr=boolean  ZeroCross=off
  Compare To Zero5 : simulink/Logic and Bit Operations/Compare To Zero  relop=<  OutDataTypeStr=boolean  ZeroCross=off
  Compare To Zero6 : simulink/Logic and Bit Operations/Compare To Zero  relop=>=  OutDataTypeStr=boolean  ZeroCross=off
  Compare To Zero7 : simulink/Logic and Bit Operations/Compare To Zero  relop=>  OutDataTypeStr=boolean  ZeroCross=off
  Constant : Constant  Value=0
  Constant1 : Constant  Value=0
  Delay{,1..3} (4 alike) : Delay  DelayLength=1  SampleTime=PI.cur.Ts
  Demux : Demux  Outputs=2
  Demux1 : Demux  Outputs=2
  Demux2 : Demux  Outputs=2
  FILTER APPROX CURRENT LOOP BW : TransferFcn  Commented=on  Numerator=Gcc_1ord.Numerator{:,:}  Denominator=Gcc_1ord.Denominator{:,:}
  Gain : Gain  Gain=PI.cur.kpd
  Gain1 : Gain  Gain=1000
  Gain2 : Gain  Gain=PI.cur.kid
  Gain3 : Gain  Gain=PI.cur.kpq
  Gain4 : Gain  Gain=PI.cur.kiq
  Gain5 : Gain  Gain=1000
  Gain6 : Gain  Gain=1/1000
  Gain7 : Gain  Gain=1/1000
  Logical Operator{,1..3} (4 alike) : Logic  Inputs=3  AllPortsSameDT=off  OutDataTypeStr=boolean
  MATLAB Function1 : MATLAB Function  TreatAsAtomicUnit=on
  MATLAB Function3 : MATLAB Function  TreatAsAtomicUnit=on
  Mux : Mux  Inputs=2
  Mux2 : Mux  Inputs=2
  NOT : Logic  Operator=NOT  AllPortsSameDT=off  OutDataTypeStr=boolean
  OR : Logic  Operator=OR  AllPortsSameDT=off  OutDataTypeStr=boolean
  OR1 : Logic  Operator=OR  AllPortsSameDT=off  OutDataTypeStr=boolean
  Scope{,1..2,7} (4 alike) : Scope  NumInputPorts=2
  Scope3 : Scope
  Scope4 : Scope
  Sum : Sum  Inputs=|+-
  Sum1 : Sum  Inputs=-+|
  Sum2 : Sum  Inputs=++|
  Sum3 : Sum  Inputs=|++
  Sum4 : Sum  Inputs=|++
  Sum5 : Sum  Inputs=|+-
  Sum6 : Sum  Inputs=|++
  Sum7 : Sum  Inputs=-+|
  Switch : Switch  Criteria=u2 > Threshold
  Switch1 : Switch  Criteria=u2 > Threshold
  Vdq* : Outport
  wires:
  Sum/1 -> Compare To Zero5/1, Compare To Zero7/1, Switch1/3, Gain/1, Scope1/2, Scope2/1
  Switch/1 -> Gain4/1, Scope/2
  MATLAB Function1/1(y) -> Scope7/2, Gain7/1, [Vq_ref]
  MATLAB Function3/1(y) -> Scope7/1, Gain6/1
  Demux/2 -> Sum1/1
  Gain2/1 -> Delay2/1
  Sum6/1 -> Sum2/1, Delay3/1
  Delay2/1 -> Sum6/1
  Delay3/1 -> Sum6/2
  Delay1/1 -> Sum4/2
  Delay/1 -> Sum4/1
  iq*/1 -> Sum7/2, Sum1/2
  Demux1/2 -> [uq_sat]
  Demux1/1 -> [ud_sat]
  udq_sat/1 -> Demux1/1
  Switch1/1 -> Gain2/1, Scope1/1
  Constant1/1 -> Switch1/1
  OR1/1 -> Switch1/2
  [satON] -> Logical Operator3/1, Logical Operator2/3
  Logical Operator2/1 -> OR1/1
  Logical Operator3/1 -> OR1/2
  Compare To Zero5/1 -> Logical Operator2/2
  Compare To Zero4/1 -> Logical Operator2/1
  Compare To Zero6/1 -> Logical Operator3/3
  [ud_sat] -> Compare To Zero6/1, Compare To Zero4/1
  Compare To Zero7/1 -> Logical Operator3/2
  Compare To Zero3/1 -> Logical Operator1/2
  [uq_sat] -> Compare To Zero/1, Compare To Zero2/1
  Compare To Zero2/1 -> Logical Operator1/3
  Compare To Zero/1 -> Logical Operator/1
  Compare To Zero1/1 -> Logical Operator/2
  Logical Operator1/1 -> OR/2
  Logical Operator/1 -> OR/1
  NOT/1 -> Switch/2
  OR/1 -> NOT/1
  Constant/1 -> Switch/3
  Gain3/1 -> Sum3/1
  Gain4/1 -> Delay/1
  Gain/1 -> Sum2/2
  Sum1/1 -> Compare To Zero1/1, Compare To Zero3/1, Gain3/1, Scope/1, Switch/1, Scope2/2
  Sum4/1 -> Sum3/2, Delay1/1
  Sum2/1 -> Mux2/1
  Sum3/1 -> Mux2/2
  Demux/1 -> Sum/2
  idq/1 -> Demux2/1, Demux/1
  satON/1 -> Logical Operator1/1, Logical Operator/3, [satON]
  Demux2/2 -> Sum7/1
  Demux2/1 -> Sum5/2
  Sum5/1 -> Scope4/1, Gain1/1
  Sum7/1 -> Gain5/1
  id*/1 -> Sum5/1, Sum/1
  Mux2/1 -> Vdq*/1, Scope3/1
  Gain1/1 -> MATLAB Function3/1(u)
  Gain5/1 -> MATLAB Function1/1(u)
  Gain6/1 -> Mux/1
  Gain7/1 -> Mux/2

== system SalientPolePMSM/FOC1/Rev_Park ==
  note: OUTPUT
  note: INPUTS
  dq : Inport
  thme : Inport  Port=2
  Add2 : Sum  Inputs=+-
  Add3 : Sum
  Cos2 : Trigonometry  Operator=cos
  Demux2 : Demux  Outputs=2
  Mux1 : Mux  Inputs=2
  Product{,1..3} (4 alike) : Product
  Sin2 : Trigonometry
  AB : Outport
  wires:
  Mux1/1 -> AB/1
  Sin2/1 -> Product1/2, Product2/2
  Demux2/2 -> Product1/1, Product3/2
  Product2/1 -> Add3/1
  Product3/1 -> Add3/2
  thme/1 -> Sin2/1, Cos2/1
  Demux2/1 -> Product2/1, Product/1
  Cos2/1 -> Product3/1, Product/2
  Product1/1 -> Add2/2
  Add3/1 -> Mux1/2
  Add2/1 -> Mux1/1
  Product/1 -> Add2/1
  dq/1 -> Demux2/1

== system SalientPolePMSM/FOC1/Rev_Park 2 ==
  note: OUTPUT
  note: INPUTS
  dq : Inport
  thme : Inport  Port=2
  Add2 : Sum
  Add3 : Sum  Inputs=+-
  Cos2 : Trigonometry  Operator=cos
  Demux2 : Demux  Outputs=2
  Gain2 : Gain  Gain=2
  Gain3 : Gain  Gain=-1/sqrt(3)
  Mux1 : Mux  Inputs=2
  Product{,1..3,5} (5 alike) : Product
  Sin2 : Trigonometry
  AB : Outport
  wires:
  Product3/1 -> Add2/1
  Demux2/2 -> Product2/1, Product3/2
  Mux1/1 -> AB/1
  Sin2/1 -> Product1/2, Product2/2
  thme/1 -> Sin2/1, Cos2/1
  Cos2/1 -> Product/2, Product3/1
  Product1/1 -> Add2/2
  dq/1 -> Demux2/1
  ? -> Gain2/1
  Product5/1 -> Gain3/1
  Gain2/1 -> Product5/2
  ? -> Product5/1
  Gain3/1 -> ?
  Add3/1 -> Mux1/2
  Add2/1 -> Mux1/1
  Product2/1 -> Add3/2
  Product/1 -> Add3/1
  Demux2/1 -> Product/1, Product1/1

== system SalientPolePMSM/FOC1/Subsystem1 ==
  note: OUTPUT
  note: INPUTS
  dq : Inport
  Demux2 : Demux  Outputs=2
  Gain : Gain  Gain=-1
  Mux1 : Mux  Inputs=2
  qd : Outport
  wires:
  Mux1/1 -> qd/1
  dq/1 -> Demux2/1
  Demux2/1 -> Mux1/2
  Demux2/2 -> Gain/1
  Gain/1 -> Mux1/1

== system SalientPolePMSM/FOC1/Subsystem4 ==
  note: OUTPUT
  note: INPUTS
  dq : Inport
  thme : Inport  Port=2
  Add2 : Sum  Inputs=+-
  Add3 : Sum
  Cos2 : Trigonometry  Operator=cos
  Demux2 : Demux  Outputs=2
  Mux1 : Mux  Inputs=2
  Product{,1..3} (4 alike) : Product
  Sin2 : Trigonometry
  AB : Outport
  wires:
  Mux1/1 -> AB/1
  Sin2/1 -> Product1/2, Product2/2
  Demux2/2 -> Product1/1, Product3/2
  Product2/1 -> Add3/1
  Product3/1 -> Add3/2
  thme/1 -> Sin2/1, Cos2/1
  Demux2/1 -> Product2/1, Product/1
  Cos2/1 -> Product3/1, Product/2
  Product1/1 -> Add2/2
  Add3/1 -> Mux1/2
  Add2/1 -> Mux1/1
  Product/1 -> Add2/1
  dq/1 -> Demux2/1

== system SalientPolePMSM/FOC2/Changed1 ==
  note: Variations
  note: INPUTS
  note: OUTPUT
  dq : Inport
  thme : Inport  Port=2
  Add2 : Sum
  Add3 : Sum  Inputs=+-
  Cos2 : Trigonometry  Operator=cos
  Demux2 : Demux  Outputs=2
  Mux1 : Mux  Inputs=2
  Product{,1..3} (4 alike) : Product
  Sin2 : Trigonometry
  Subsystem : Subsystem
  AB : Outport
  wires:
  Product3/1 -> Add2/1
  Demux2/2 -> Product2/1, Product3/2
  Demux2/1 -> Product/1, Product1/1
  Mux1/1 -> AB/1
  Sin2/1 -> Product1/2, Product2/2
  thme/1 -> Sin2/1, Cos2/1
  Cos2/1 -> Product3/1, Product/2
  Product1/1 -> Add2/2
  dq/1 -> Demux2/1
  Add3/1 -> Mux1/2
  Add2/1 -> Mux1/1
  Product2/1 -> Add3/2
  Product/1 -> Add3/1

== system SalientPolePMSM/FOC2/Circle Limitation ==
  dq : Inport
  Demux : Demux  Outputs=2
  Gain : Gain  Gain=1000
  Gain1 : Gain  Gain=1000
  Gain2 : Gain  Gain=1/1000
  Gain3 : Gain  Gain=1/1000
  MATLAB Function : MATLAB Function  TreatAsAtomicUnit=on
  Mux : Mux  Inputs=2
  dq* : Outport
  wires:
  Demux/2 -> Gain1/1
  Demux/1 -> Gain/1
  Mux/1 -> dq*/1
  dq/1 -> Demux/1
  MATLAB Function/1(new_d) -> Gain2/1
  MATLAB Function/2(new_q) -> Gain3/1
  Gain2/1 -> Mux/1
  Gain3/1 -> Mux/2
  Gain/1 -> MATLAB Function/1(u_d)
  Gain1/1 -> MATLAB Function/2(u_q)

== system SalientPolePMSM/FOC2/Decoupling1 ==
  note: INPUTS:
  note: OUTPUT:
  udq* : Inport
  idq : Inport  Port=2
  wme : Inport  Port=3
  Demux : Demux  Outputs=2
  Demux1 : Demux  Outputs=2
  Demux2 : Demux  Outputs=2
  Gain : Gain  Gain=PI.cur.Ld
  Gain1 : Gain  Gain=PI.cur.Lq
  Gain2 : Gain  Gain=PI.cur.lammg
  Mux : Mux  Inputs=2
  Product : Product
  Product1 : Product
  Scope : Scope
  Scope1 : Scope
  Subtract : Sum  Inputs=-+
  Subtract1 : Sum  Inputs=+++
  Terminator1 : Terminator
  Terminator4 : Terminator
  idq1 : InportShadow  Port=2
  wme1 : InportShadow  Port=3
  udq** : Outport
  wires:
  Product1/1 -> Scope/1, Subtract/1  "wme*iq*Lq"
  wme1/1 -> Gain1/1
  Gain1/1 -> Product1/2
  Demux1/1 -> Terminator4/1
  idq1/1 -> Demux1/1
  Demux1/2 -> Product1/1  "iq"
  udq*/1 -> Demux/1
  Mux/1 -> udq**/1
  Gain/1 -> Product/1
  Gain2/1 -> Subtract1/2  "wme*lammg"
  Subtract1/1 -> Mux/2
  wme/1 -> Gain2/1, Gain/1
  Demux/1 -> Subtract/2
  Demux2/2 -> Terminator1/1
  Demux/2 -> Subtract1/1
  Subtract/1 -> Mux/1
  Product/1 -> Subtract1/3  "wme*id*Ld"
  idq/1 -> Demux2/1, Scope1/1
  Demux2/1 -> Product/2  "id"

== system SalientPolePMSM/FOC2/Decoupling2 ==
  note: INPUTS:
  note: OUTPUT:
  udq* : Inport
  idq : Inport  Port=2
  wme : Inport  Port=3
  Demux : Demux  Outputs=2
  Demux1 : Demux  Outputs=2
  Demux2 : Demux  Outputs=2
  Gain : Gain  Gain=PI.cur.Ld
  Gain1 : Gain  Gain=PI.cur.Lq
  Gain2 : Gain  Gain=PI.cur.lammg
  Mux : Mux  Inputs=2
  Product : Product
  Product1 : Product
  Scope : Scope
  Scope1 : Scope
  Subtract : Sum  Inputs=-+
  Subtract1 : Sum  Inputs=+++
  Terminator1 : Terminator
  Terminator4 : Terminator
  idq1 : InportShadow  Port=2
  wme1 : InportShadow  Port=3
  udq** : Outport
  wires:
  Product1/1 -> Scope/1, Subtract/1  "wme*iq*Lq"
  wme1/1 -> Gain1/1
  Gain1/1 -> Product1/2
  Demux1/1 -> Terminator4/1
  idq1/1 -> Demux1/1
  Demux1/2 -> Product1/1  "iq"
  udq*/1 -> Demux/1
  Mux/1 -> udq**/1
  Gain/1 -> Product/1
  Gain2/1 -> Subtract1/2  "wme*lammg"
  Subtract1/1 -> Mux/2
  wme/1 -> Gain2/1, Gain/1
  Demux/1 -> Subtract/2
  Demux2/2 -> Terminator1/1
  Demux/2 -> Subtract1/1
  Subtract/1 -> Mux/1
  Product/1 -> Subtract1/3  "wme*id*Ld"
  idq/1 -> Demux2/1, Scope1/1
  Demux2/1 -> Product/2  "id"

== system SalientPolePMSM/FOC2/INVERTER1 ==
  note: OUTPUTS:
  note: INPUTS:
  uAB : Inport
  uBus : Inport  Port=2
  iabc : Inport  Port=3
  INVERTER power driver : Subsystem
  SVM algorithm : Subsystem
  Scope : Scope
  uabc_n* : Outport
  uabc_n*nonideal : Outport  Port=2
  satON : Outport  Port=3
  wires:
  INVERTER power driver/1(uabc_n*) -> uabc_n*/1
  uAB/1 -> SVM algorithm/1(UABref)
  INVERTER power driver/2(uabc_n*nonideal) -> uabc_n*nonideal/1
  iabc/1 -> INVERTER power driver/3(iabc)
  SVM algorithm/1(duties) -> INVERTER power driver/1(duties), Scope/1  "duties"
  [satON] -> satON/1
  SVM algorithm/2(satON) -> [satON]
  uBus/1 -> INVERTER power driver/2(uBus), SVM algorithm/2(uBus)

== system SalientPolePMSM/FOC2/INVERTER2 ==
  note: OUTPUTS:
  note: INPUTS:
  uAB : Inport
  uBus : Inport  Port=2
  iabc : Inport  Port=3
  INVERTER power driver : Subsystem
  SVM algorithm : Subsystem
  Scope : Scope  NumInputPorts=2
  Scope1 : Scope
  uabc_n* : Outport
  uabc_n*nonideal : Outport  Port=2
  satON : Outport  Port=3
  wires:
  INVERTER power driver/2(uabc_n*nonideal) -> uabc_n*nonideal/1
  iabc/1 -> INVERTER power driver/3(iabc)
  SVM algorithm/1(duties) -> Scope/1, INVERTER power driver/1(duties)  "duties"
  [satON] -> satON/1
  uBus/1 -> INVERTER power driver/2(uBus), SVM algorithm/2(uBus)
  uAB/1 -> Scope1/1, SVM algorithm/1(VABref)
  INVERTER power driver/1(uabc_n*) -> Scope/2, uabc_n*/1

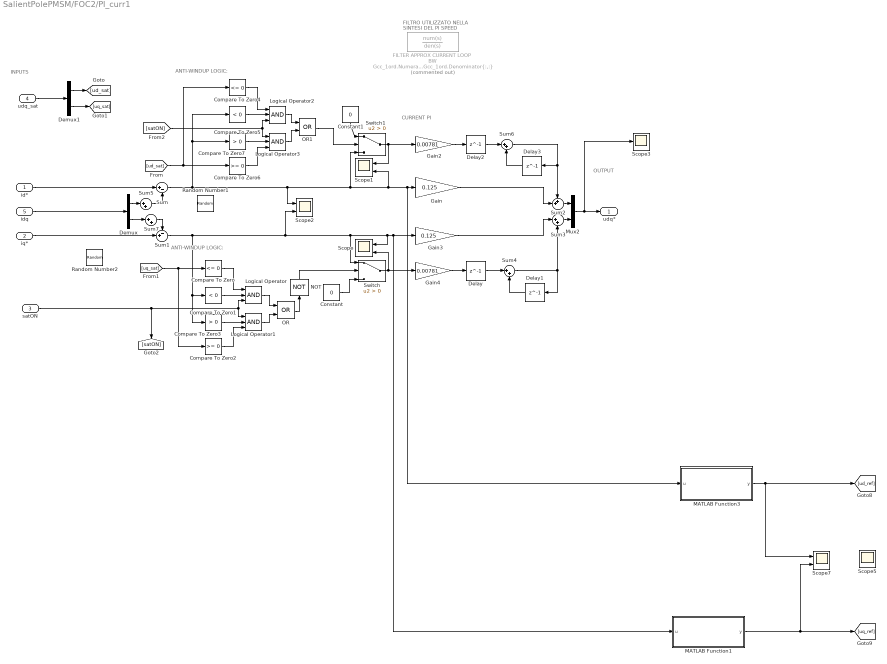
== system SalientPolePMSM/FOC2/PI_curr1 ==
  note: INPUTS
  note: OUTPUT
  note: ANTI-WINDUP LOGIC:
  note: ANTI-WINDUP LOGIC:
  note: CURRENT PI
  note: FILTRO UTILIZZATO
      | NELLA SINTESI DEL
      | PI SPEED
  id* : Inport
  iq* : Inport  Port=2
  satON : Inport  Port=3
  udq_sat : Inport  Port=4
  idq : Inport  Port=5
  Compare To Zero : simulink/Logic and Bit Operations/Compare To Zero  relop=<=  OutDataTypeStr=boolean  ZeroCross=off
  Compare To Zero1 : simulink/Logic and Bit Operations/Compare To Zero  relop=<  OutDataTypeStr=boolean  ZeroCross=off
  Compare To Zero2 : simulink/Logic and Bit Operations/Compare To Zero  relop=>=  OutDataTypeStr=boolean  ZeroCross=off
  Compare To Zero3 : simulink/Logic and Bit Operations/Compare To Zero  relop=>  OutDataTypeStr=boolean  ZeroCross=off
  Compare To Zero4 : simulink/Logic and Bit Operations/Compare To Zero  relop=<=  OutDataTypeStr=boolean  ZeroCross=off
  Compare To Zero5 : simulink/Logic and Bit Operations/Compare To Zero  relop=<  OutDataTypeStr=boolean  ZeroCross=off
  Compare To Zero6 : simulink/Logic and Bit Operations/Compare To Zero  relop=>=  OutDataTypeStr=boolean  ZeroCross=off
  Compare To Zero7 : simulink/Logic and Bit Operations/Compare To Zero  relop=>  OutDataTypeStr=boolean  ZeroCross=off
  Constant : Constant  Value=0
  Constant1 : Constant  Value=0
  Delay{,1..3} (4 alike) : Delay  DelayLength=1  SampleTime=PI.cur.Ts
  Demux : Demux  Outputs=2
  Demux1 : Demux  Outputs=2
  FILTER APPROX CURRENT LOOP BW : TransferFcn  Commented=on  Numerator=Gcc_1ord.Numerator{:,:}  Denominator=Gcc_1ord.Denominator{:,:}
  Gain : Gain  Gain=0.125
  Gain2 : Gain  Gain=0.00781
  Gain3 : Gain  Gain=0.125
  Gain4 : Gain  Gain=0.00781
  Logical Operator{,1..3} (4 alike) : Logic  Inputs=3  AllPortsSameDT=off  OutDataTypeStr=boolean
  MATLAB Function1 : MATLAB Function  TreatAsAtomicUnit=on
  MATLAB Function3 : MATLAB Function  TreatAsAtomicUnit=on
  Mux2 : Mux  Inputs=2
  NOT : Logic  Operator=NOT  AllPortsSameDT=off  OutDataTypeStr=boolean
  OR : Logic  Operator=OR  AllPortsSameDT=off  OutDataTypeStr=boolean
  OR1 : Logic  Operator=OR  AllPortsSameDT=off  OutDataTypeStr=boolean
  Random Number1 : RandomNumber  Variance=0.01  SampleTime=inv.Ts
  Random Number2 : RandomNumber  Variance=0.125  SampleTime=inv.Ts
  Scope{,1..2,7} (4 alike) : Scope  NumInputPorts=2
  Scope3 : Scope
  Scope5 : Scope
  Sum : Sum  Inputs=|+-
  Sum1 : Sum  Inputs=-+|
  Sum2 : Sum  Inputs=++|
  Sum{3..7} (5 alike) : Sum  Inputs=|++
  Switch : Switch  Criteria=u2 > Threshold
  Switch1 : Switch  Criteria=u2 > Threshold
  udq* : Outport
  wires:
  Sum/1 -> Compare To Zero5/1, Compare To Zero7/1, Switch1/3, Gain/1, MATLAB Function3/1(u), Scope1/2, Scope2/1
  Switch/1 -> Gain4/1, Scope/2
  MATLAB Function1/1(y) -> Scope7/2, [uq_ref]
  MATLAB Function3/1(y) -> [ud_ref], Scope7/1
  Sum7/1 -> Sum1/1
  Demux/2 -> Sum7/1
  Demux/1 -> Sum5/1
  Sum5/1 -> Sum/2
  Gain2/1 -> Delay2/1
  Sum6/1 -> Sum2/1, Delay3/1
  Delay2/1 -> Sum6/1
  Delay3/1 -> Sum6/2
  Delay1/1 -> Sum4/2
  Delay/1 -> Sum4/1
  iq*/1 -> Sum1/2
  Demux1/2 -> [uq_sat]
  Demux1/1 -> [ud_sat]
  udq_sat/1 -> Demux1/1
  Switch1/1 -> Gain2/1, Scope1/1
  Constant1/1 -> Switch1/1
  OR1/1 -> Switch1/2
  [satON] -> Logical Operator3/1, Logical Operator2/3
  Logical Operator2/1 -> OR1/1
  Logical Operator3/1 -> OR1/2
  Compare To Zero5/1 -> Logical Operator2/2
  Compare To Zero4/1 -> Logical Operator2/1
  Compare To Zero6/1 -> Logical Operator3/3
  [ud_sat] -> Compare To Zero6/1, Compare To Zero4/1
  Compare To Zero7/1 -> Logical Operator3/2
  Compare To Zero3/1 -> Logical Operator1/2
  [uq_sat] -> Compare To Zero/1, Compare To Zero2/1
  Compare To Zero2/1 -> Logical Operator1/3
  Compare To Zero/1 -> Logical Operator/1
  Compare To Zero1/1 -> Logical Operator/2
  Logical Operator1/1 -> OR/2
  Logical Operator/1 -> OR/1
  satON/1 -> Logical Operator1/1, Logical Operator/3, [satON]
  NOT/1 -> Switch/2
  OR/1 -> NOT/1
  Constant/1 -> Switch/3
  id*/1 -> Sum/1
  idq/1 -> Demux/1
  Gain3/1 -> Sum3/1
  Gain4/1 -> Delay/1
  Gain/1 -> Sum2/2
  Sum1/1 -> Compare To Zero1/1, Compare To Zero3/1, Gain3/1, MATLAB Function1/1(u), Scope/1, Switch/1, Scope2/2
  Sum4/1 -> Sum3/2, Delay1/1
  Sum2/1 -> Mux2/1
  Sum3/1 -> Mux2/2
  Mux2/1 -> udq*/1, Scope3/1
